simulink subsystem "vehicle_dynamics_old"  (R2022a)
settings: Solver=VariableStepAuto  StartTime=0.0  StopTime=10.0  RelTol=1e-3
undefined symbols (not defined in the file): DiscIntNeverNeededParam, pac, param, vx0, vy0, wFL0, wFR0, wRL0, wRR0, yaw_rate0
settings Model: Creator=jutri  LastModifiedBy=Usuario
settings ModelReferenceCC: EnableRefExpFcnMdlSchedulingChecks=off
settings RTWCC: Description=Generic Real-Time Target  GPUComputeCapability=5.0

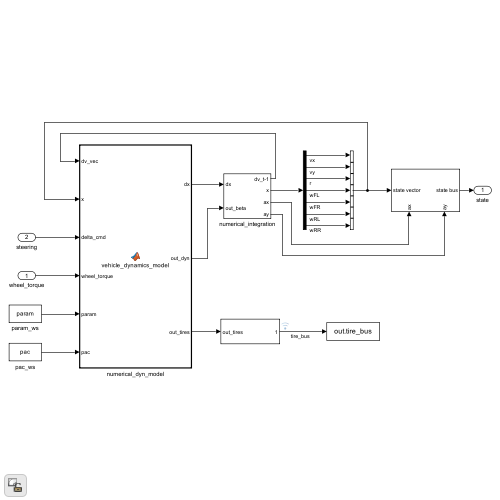
[thumbnail: Simulink's stored preview of the top-level diagram]
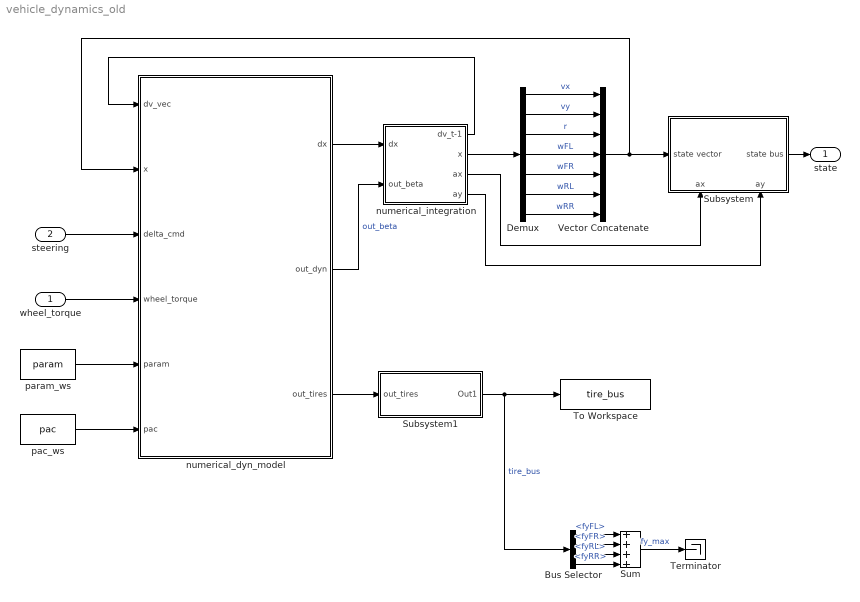
== system vehicle_dynamics_old ==
  wheel_torque : Inport
  steering : Inport  Port=2
  Bus Selector : BusSelector  OutputSignals=fyFL,fyFR,fyRL,fyRR
  Demux : Demux  Outputs=7
  Subsystem : Subsystem
      settings: PortSchema="{\"entries\":[{\"content\":{\"sides\":[{\"content\":{\"connectorIds\":[\"In1\"]},\"type\":\"ConnectorPlacement.EquallySpacedRectSide\",\"uuid\":\"722aa60e-e1ec-43eb-b2d5-2e5609c6fcbb\"},{\"content\":{\"connectorIds\":[\"Out1\"],\"side\":\"RIGHT\"},\"type\":\"ConnectorPlacement.EquallySpacedRectSide\",\"uuid\":\"c719093c-3553-44fc-93c2-7bf8d353ce79\"},{\"content\":{\"side\":\"TOP\"},\"type\":\"ConnectorPlacement.EquallySpacedRectSide\",\"uuid\":\"e7bb3d1e-0d92-481c-a4d7-3f96134ca887\"},{\"content\":{\"connectorIds\":[\"In2\",\"In3\"],\"side\":\"BOTTOM\"},\"type\":\"ConnectorPlacement.EquallySpacedRectSide\",\"uuid\":\"ef1ebdd3-6d45-4770-b9ab-304fa76891a1\"}]},\"type\":\"ConnectorPlacement.EquallySpacedConnector\",\"uuid\":\"5fd2dd50-6bec-4848-93bb-31d640afba49\"}],\"packageUris\":[\"http://schema.mathworks.com/mf0/Connector/R2020b\"],\"version\":\"1.0\"}"
  Subsystem1 : Subsystem
  Sum : Sum  Inputs=++++
  Terminator : Terminator
  To Workspace : ToWorkspace  VariableName=tire_bus  SaveFormat=Structure  SampleTime=-1
  Vector Concatenate : Concatenate  NumInputs=7
  numerical_dyn_model : MATLAB Function  TreatAsAtomicUnit=on
  numerical_integration : Subsystem
  pac_ws : Constant  Value=pac  OutDataTypeStr=Bus: pacBus
  param_ws : Constant  Value=param  OutDataTypeStr=Bus: paramBus
  state : Outport
  wires:
  steering/1 -> numerical_dyn_model/3(delta_cmd)
  numerical_dyn_model/1(dx) -> numerical_integration/1(dx)
  wheel_torque/1 -> numerical_dyn_model/4(wheel_torque)
  numerical_integration/2(x) -> Demux/1
  param_ws/1 -> numerical_dyn_model/5(param)
  Subsystem/1(state bus) -> state/1
  pac_ws/1 -> numerical_dyn_model/6(pac)
  numerical_integration/3(ax) -> Subsystem/2(ax)
  numerical_integration/4(ay) -> Subsystem/3(ay)
  numerical_integration/1(dv_t-1) -> numerical_dyn_model/1(dv_vec)
  Demux/1 -> Vector Concatenate/1  "vx"
  Demux/2 -> Vector Concatenate/2  "vy"
  Demux/3 -> Vector Concatenate/3  "r"
  Demux/4 -> Vector Concatenate/4  "wFL"
  Demux/5 -> Vector Concatenate/5  "wFR"
  Demux/6 -> Vector Concatenate/6  "wRL"
  Demux/7 -> Vector Concatenate/7  "wRR"
  Vector Concatenate/1 -> numerical_dyn_model/2(x), Subsystem/1(state vector)
  numerical_dyn_model/2(out_dyn) -> numerical_integration/2(out_beta)  "out_beta"
  Subsystem1/1(Out1) -> To Workspace/1, Bus Selector/1  "tire_bus"
  numerical_dyn_model/3(out_tires) -> Subsystem1/1(out_tires)
  Bus Selector/1 -> Sum/1  "<fyFL>"
  Bus Selector/2 -> Sum/2  "<fyFR>"
  Bus Selector/3 -> Sum/3  "<fyRL>"
  Bus Selector/4 -> Sum/4  "<fyRR>"
  Sum/1 -> Terminator/1  "fy_max"

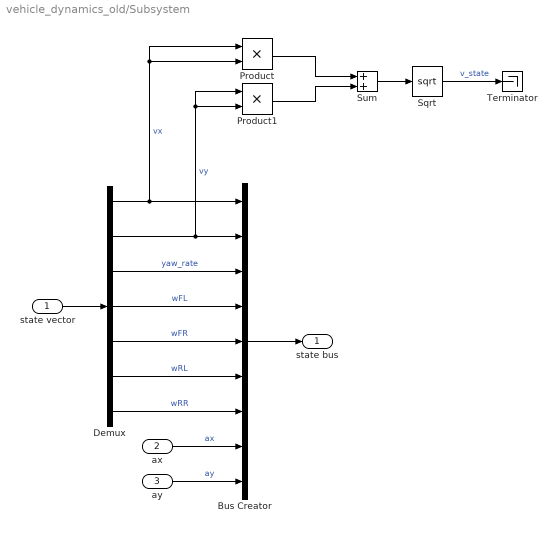
== system vehicle_dynamics_old/Subsystem ==
  state vector : Inport
  ax : Inport  Port=2
  ay : Inport  Port=3
  Bus Creator : BusCreator  Inputs=9
  Demux : Demux  Outputs=7
  Product : Product
  Product1 : Product
  Sqrt : Sqrt
  Sum : Sum
  Terminator : Terminator
  state bus : Outport
  wires:
  Sqrt/1 -> Terminator/1  "v_state"
  Sum/1 -> Sqrt/1
  Product/1 -> Sum/1
  Product1/1 -> Sum/2
  Bus Creator/1 -> state bus/1
  ay/1 -> Bus Creator/9  "ay"
  ax/1 -> Bus Creator/8  "ax"
  Demux/7 -> Bus Creator/7  "wRR"
  Demux/6 -> Bus Creator/6  "wRL"
  Demux/2 -> Bus Creator/2, Product1/1, Product1/2  "vy"
  Demux/3 -> Bus Creator/3  "yaw_rate"
  Demux/1 -> Bus Creator/1, Product/1, Product/2  "vx"
  Demux/4 -> Bus Creator/4  "wFL"
  Demux/5 -> Bus Creator/5  "wFR"
  state vector/1 -> Demux/1

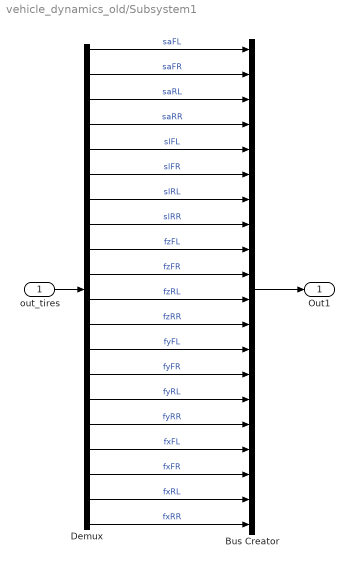
== system vehicle_dynamics_old/Subsystem1 ==
  out_tires : Inport
  Bus Creator : BusCreator  Inputs=20
  Demux : Demux  Outputs=20
  Out1 : Outport
  wires:
  Bus Creator/1 -> Out1/1
  Demux/20 -> Bus Creator/20  "fxRR"
  Demux/19 -> Bus Creator/19  "fxRL"
  Demux/18 -> Bus Creator/18  "fxFR"
  Demux/17 -> Bus Creator/17  "fxFL"
  Demux/16 -> Bus Creator/16  "fyRR"
  Demux/15 -> Bus Creator/15  "fyRL"
  Demux/14 -> Bus Creator/14  "fyFR"
  Demux/13 -> Bus Creator/13  "fyFL"
  Demux/12 -> Bus Creator/12  "fzRR"
  Demux/11 -> Bus Creator/11  "fzRL"
  Demux/10 -> Bus Creator/10  "fzFR"
  Demux/9 -> Bus Creator/9  "fzFL"
  Demux/8 -> Bus Creator/8  "slRR"
  Demux/7 -> Bus Creator/7  "slRL"
  Demux/6 -> Bus Creator/6  "slFR"
  Demux/5 -> Bus Creator/5  "slFL"
  Demux/4 -> Bus Creator/4  "saRR"
  Demux/3 -> Bus Creator/3  "saRL"
  Demux/2 -> Bus Creator/2  "saFR"
  Demux/1 -> Bus Creator/1  "saFL"
  out_tires/1 -> Demux/1

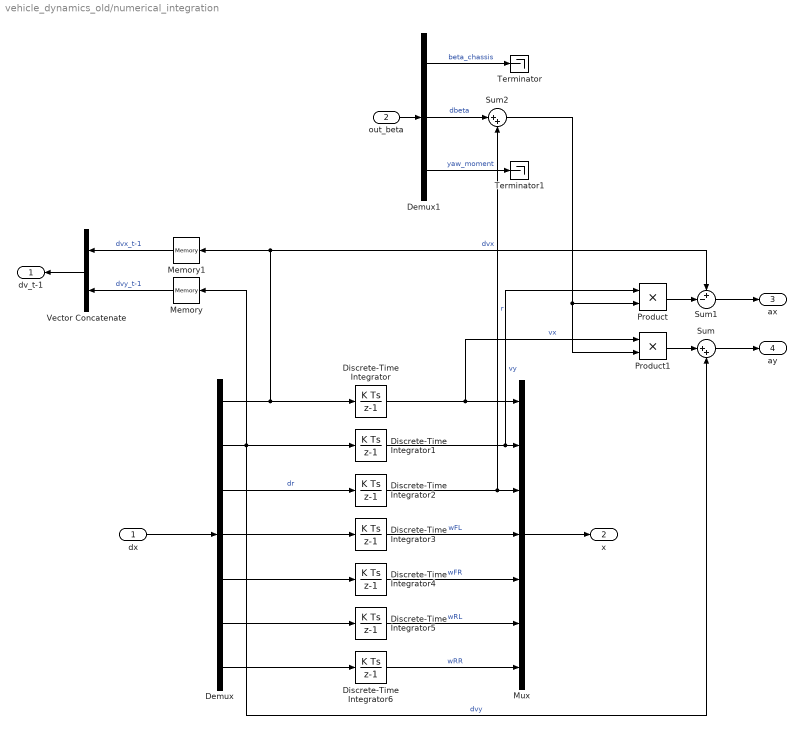
== system vehicle_dynamics_old/numerical_integration ==
  dx : Inport
  out_beta : Inport  Port=2
  Demux : Demux  Outputs=7
  Demux1 : Demux  Outputs=3
  Discrete-Time Integrator : DiscreteIntegrator  InitialCondition=vx0  SampleTime=-1  ICPrevOutput=DiscIntNeverNeededParam  ICPrevScaledInput=DiscIntNeverNeededParam
  Discrete-Time Integrator1 : DiscreteIntegrator  InitialCondition=vy0  SampleTime=-1  ICPrevOutput=DiscIntNeverNeededParam  ICPrevScaledInput=DiscIntNeverNeededParam
  Discrete-Time Integrator2 : DiscreteIntegrator  InitialCondition=yaw_rate0  SampleTime=-1  ICPrevOutput=DiscIntNeverNeededParam  ICPrevScaledInput=DiscIntNeverNeededParam
  Discrete-Time Integrator3 : DiscreteIntegrator  InitialCondition=wFL0  SampleTime=-1  ICPrevOutput=DiscIntNeverNeededParam  ICPrevScaledInput=DiscIntNeverNeededParam
  Discrete-Time Integrator4 : DiscreteIntegrator  InitialCondition=wFR0  SampleTime=-1  ICPrevOutput=DiscIntNeverNeededParam  ICPrevScaledInput=DiscIntNeverNeededParam
  Discrete-Time Integrator5 : DiscreteIntegrator  InitialCondition=wRL0  SampleTime=-1  ICPrevOutput=DiscIntNeverNeededParam  ICPrevScaledInput=DiscIntNeverNeededParam
  Discrete-Time Integrator6 : DiscreteIntegrator  InitialCondition=wRR0  SampleTime=-1  ICPrevOutput=DiscIntNeverNeededParam  ICPrevScaledInput=DiscIntNeverNeededParam
  Memory : Memory
  Memory1 : Memory
  Mux : Mux  Inputs=7
  Product : Product
  Product1 : Product
  Sum : Sum  Inputs=|++
  Sum1 : Sum  Inputs=+-|
  Sum2 : Sum  Inputs=|++
  Terminator : Terminator
  Terminator1 : Terminator
  Vector Concatenate : Concatenate
  dv_t-1 : Outport
  x : Outport  Port=2
  ax : Outport  Port=3
  ay : Outport  Port=4
  wires:
  Demux1/3 -> Terminator1/1  "yaw_moment"
  Sum2/1 -> Product/2, Product1/2
  Demux1/2 -> Sum2/1  "dbeta"
  Demux1/1 -> Terminator/1  "beta_chassis"
  out_beta/1 -> Demux1/1
  Sum1/1 -> ax/1
  Product/1 -> Sum1/2
  Sum/1 -> ay/1
  Product1/1 -> Sum/1
  Vector Concatenate/1 -> dv_t-1/1
  Memory/1 -> Vector Concatenate/2  "dvy_t-1"
  Memory1/1 -> Vector Concatenate/1  "dvx_t-1"
  Discrete-Time Integrator3/1 -> Mux/4  "wFL"
  Discrete-Time Integrator6/1 -> Mux/7  "wRR"
  Discrete-Time Integrator5/1 -> Mux/6  "wRL"
  Discrete-Time Integrator4/1 -> Mux/5  "wFR"
  Demux/4 -> Discrete-Time Integrator3/1
  Demux/5 -> Discrete-Time Integrator4/1
  Demux/6 -> Discrete-Time Integrator5/1
  Demux/7 -> Discrete-Time Integrator6/1
  Discrete-Time Integrator2/1 -> Sum2/2, Mux/3  "r"
  Demux/3 -> Discrete-Time Integrator2/1  "dr"
  Discrete-Time Integrator1/1 -> Mux/2, Product/1  "vy"
  Demux/2 -> Sum/2, Memory/1, Discrete-Time Integrator1/1  "dvy"
  Discrete-Time Integrator/1 -> Mux/1, Product1/1  "vx"
  Demux/1 -> Discrete-Time Integrator/1, Sum1/1, Memory1/1  "dvx"
  Mux/1 -> x/1
  dx/1 -> Demux/1

== matlab function vehicle_dynamics_old/numerical_dyn_model ==
  data: dv_vec input; x input; delta_cmd input; dx output; out_dyn output; wheel_torque input; param input; pac input; out_tires output
function [dx, out_dyn, out_tires] = vehicle_dynamics_model(dv_vec, x, delta_cmd, wheel_torque, param,pac)

% Nonlinear vehicle model
%   Input: u = [delta_cmd, wheel_torque]
%   State: 7x1  x
%       x(1) = vx [m/s]
%       x(2) = vy [m/s]
%       x(3) = yaw_rate [rad/s]
%       x(4) = wheel_speed_FL [rad/s]
%       x(5) = wheel_speed_FR [rad/s]
%       x(6) = wheel_speed_RL [rad/s]
%       x(7) = wheel_speed_RR [rad/s]

dx = zeros(7,1);

%% Initial state
vx = x(1);
vy = x(2);
yaw_rate = x(3);
wheel_speed = x(4:7);

beta = atan(vy/(vx + eps));
dvx = dv_vec(1);
dvy = dv_vec(2);
d_beta = 0*1/(1+(vy/(vx+eps))^2) * (dvx*vx - dvy*vy)/ (vx^2+eps);

ax = dvx - vy * (yaw_rate + d_beta);
ay = dvy + vx * (yaw_rate + d_beta);

%% Tire calculations

delta = calculate_steering(delta_cmd, param);

vx_wheel = vx * ones(4,1) + yaw_rate / 2 * [-param.trackwidthF; param.trackwidthF; -param.trackwidthR; param.trackwidthR];
vy_wheel = vy * ones(4,1) + yaw_rate * [param.lf; param.lf; -param.lr; -param.lr];

vx_wheel_tire = vx_wheel .* cos(delta) + vy_wheel .* sin(delta);

slip_angle = atan2(vy_wheel, vx_wheel) - delta;
slip_ratio = param.rdyn * wheel_speed ./ (vx_wheel_tire + eps) - 1;

tire_load = calculate_tire_loads(ax,ay,vx,param);
[force_fy_tires, force_fx_tires] = calculate_tire_forces(tire_load,slip_angle, slip_ratio,pac);

force_fx = force_fx_tires .* cos(delta) - force_fy_tires .* sin(delta);
force_fy = force_fx_tires .* sin(delta) + force_fy_tires .* cos(delta);

fx_total = sum(force_fx) - 0.5*param.rho*param.CDA*vx^2;
yaw_moment = (force_fy(1) + force_fy(2)) * param.lf ...
            - (force_fy(3) + force_fy(4)) * param.lr ...
            + (force_fx(2) - force_fx(1))* param.trackwidthF / 2 ...
            + (force_fx(4) - force_fx(3))* param.trackwidthR / 2;

%% ODE definition

dx(1) = fx_total / param.mass + yaw_rate * vy;
dx(2) = sum(force_fy) / param.mass - yaw_rate * vx;
dx(3) = yaw_moment / param.Iz;

dx(4) = (wheel_torque(1) - param.rdyn*force_fx_tires(1)) / param.wheel_inertia;
dx(5) = (wheel_torque(2) - param.rdyn*force_fx_tires(2)) / param.wheel_inertia;
dx(6) = (wheel_torque(3) - param.rdyn*force_fx_tires(3)) / param.wheel_inertia;
dx(7) = (wheel_torque(4) - param.rdyn*force_fx_tires(4)) / param.wheel_inertia;

%% Internal state logging

out_tires = [slip_angle; slip_ratio; tire_load; force_fy_tires; force_fx_tires];

out_dyn = [beta; d_beta; yaw_moment];
